simulink model "proyectomodelado"  (R2023a)
settings: Solver=ode15s  StartTime=0.0  StopTime=5.0  RelTol=1e-3
libraries: fl_lib x14, nesl_utility x6, slpidlib x1
settings Model: Creator=yosel  LastModifiedBy=nicol
settings DataIOCC: ReturnWorkspaceOutputs=off  TimeSaveName=t
settings DebuggingCC: AlgebraicLoopMsg=none

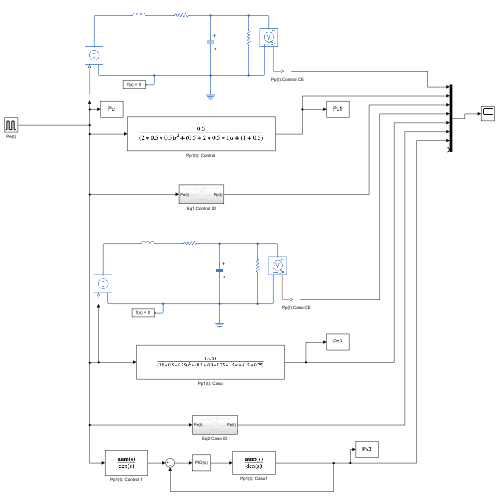
[thumbnail: Simulink's stored preview of the top-level diagram]
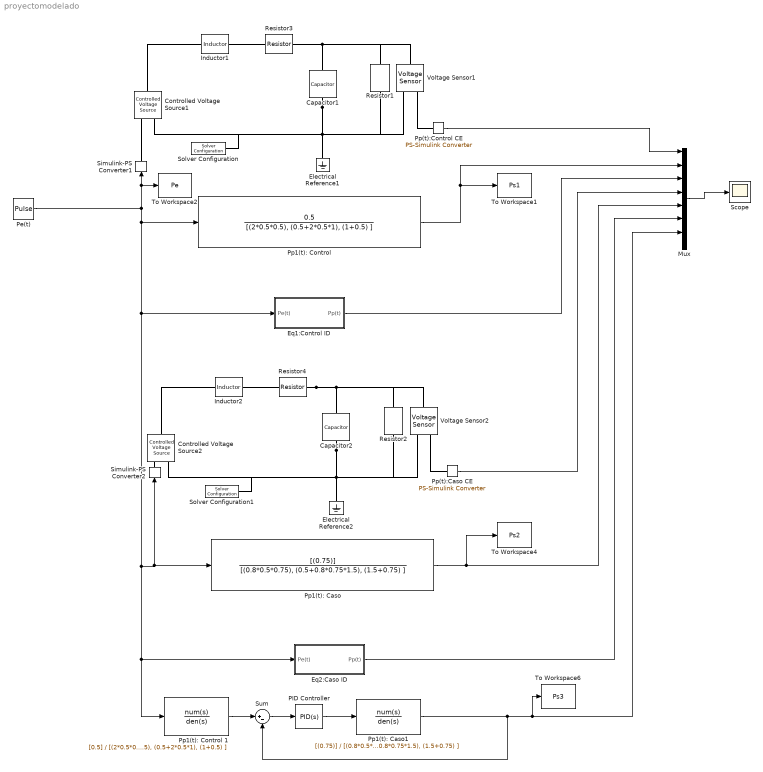
== system proyectomodelado ==
  Capacitor1 : fl_lib/Electrical/Electrical Elements/Capacitor  c=2 F  r=1e-6 Ohm  g=0 1/Ohm  i_specify=off  i_priority=None  i=0 A  i_nominal_specify=off  i_nominal_unit=A  i_nominal_value=1  v_specify=off  v_priority=None  v=0 V  v_nominal_specify=off  v_nominal_unit=V  v_nominal_value=1  vc_specify=off  vc_priority=High  vc=0 V  vc_nominal_specify=off  vc_nominal_unit=V  vc_nominal_value=1
  Capacitor2 : fl_lib/Electrical/Electrical Elements/Capacitor  c=0.8 F  r=1e-6 Ohm  g=0 1/Ohm  i_specify=off  i_priority=None  i=0 A  i_nominal_specify=off  i_nominal_unit=A  i_nominal_value=1  v_specify=off  v_priority=None  v=0 V  v_nominal_specify=off  v_nominal_unit=V  v_nominal_value=1  vc_specify=off  vc_priority=High  vc=0 V  vc_nominal_specify=off  vc_nominal_unit=V  vc_nominal_value=1
  Controlled Voltage Source1 : fl_lib/Electrical/Electrical Sources/Controlled Voltage Source
  Controlled Voltage Source2 : fl_lib/Electrical/Electrical Sources/Controlled Voltage Source
  Electrical Reference1 : fl_lib/Electrical/Electrical Elements/Electrical Reference
  Electrical Reference2 : fl_lib/Electrical/Electrical Elements/Electrical Reference
  Eq1:Control ID : Subsystem
  Eq2:Caso ID : Subsystem
  Inductor1 : fl_lib/Electrical/Electrical Elements/Inductor  l=0.5 H  r=0 Ohm  g=1e-9 1/Ohm  i_specify=off  i_priority=None  i=0 A  i_nominal_specify=off  i_nominal_unit=A  i_nominal_value=1  v_specify=off  v_priority=None  v=0 V  v_nominal_specify=off  v_nominal_unit=V  v_nominal_value=1  i_L_specify=off  i_L_priority=High  i_L=0 A  i_L_nominal_specify=off  i_L_nominal_unit=A  i_L_nominal_value=1
  Inductor2 : fl_lib/Electrical/Electrical Elements/Inductor  l=0.5 H  r=0 Ohm  g=1e-9 1/Ohm  i_specify=off  i_priority=None  i=0 A  i_nominal_specify=off  i_nominal_unit=A  i_nominal_value=1  v_specify=off  v_priority=None  v=0 V  v_nominal_specify=off  v_nominal_unit=V  v_nominal_value=1  i_L_specify=off  i_L_priority=High  i_L=0 A  i_L_nominal_specify=off  i_L_nominal_unit=A  i_L_nominal_value=1
  Mux : Mux  Inputs=8
  PID Controller : slpidlib/PID Controller  Controller=PID  Form=Parallel  TimeDomain=Continuous-time  UseExternalTs=off  SampleTime=-1  IntegratorMethod=Forward Euler  FilterMethod=Forward Euler  ControllerParametersSource=internal  P=2417168.60686299  I=213970849.102976  UseKiTs=off  D=6067.08740440942  N=1734073.08212751  UseFilter=on  TunerSelectOption=Transfer Function Based (PID Tuner App)  InitialConditionSource=internal  InitialConditionForIntegrator=0  InitialConditionForFilter=0  DifferentiatorICPrevScaledInput=0  ExternalReset=none  TrackingMode=off  Kt=1  LimitOutput=off  SatLimitsSource=internal  UpperSaturationLimit=inf  LowerSaturationLimit=-inf  LinearizeAsGain=on  AntiWindupMode=none  Kb=1  LimitIntegrator=off  UpperIntegratorSaturationLimit=inf  LowerIntegratorSaturationLimit=-inf  POutMin=[]  POutMax=[]  IOutMin=[]  IOutMax=[]  DOutMin=[]  DOutMax=[]  NOutMin=[]  NOutMax=[]  SumOutMin=[]  SumOutMax=[]  SaturationOutMin=[]  SaturationOutMax=[]  PParamMin=[]  PParamMax=[]  IParamMin=[]  IParamMax=[]  DParamMin=[]  DParamMax=[]  NParamMin=[]  NParamMax=[]  KbParamMin=[]  KbParamMax=[]  KtParamMin=[]  KtParamMax=[]  KbOutMin=[]  KbOutMax=[]  KtOutMin=[]  KtOutMax=[]  IntegratorOutMin=[]  IntegratorOutMax=[]  FilterOutMin=[]  FilterOutMax=[]  SumI1OutMin=[]  SumI1OutMax=[]  SumI2OutMin=[]  SumI2OutMax=[]  SumI3OutMin=[]  SumI3OutMax=[]  SumI4OutMin=[]  SumI4OutMax=[]  SumDOutMin=[]  SumDOutMax=[]  DifferentiatorOutMin=[]  DifferentiatorOutMax=[]  FilterDiffOutCoefMin=[]  FilterDiffOutCoefMax=[]  ReciprocalOutMin=[]  ReciprocalOutMax=[]  SumDenOutMin=[]  SumDenOutMax=[]  SumNumOutMin=[]  SumNumOutMax=[]  DivideOutMin=[]  DivideOutMax=[]  UdiffTsProdOutMin=[]  UdiffTsProdOutMax=[]  NTsProdOutMin=[]  NTsProdOutMax=[]  UintegralTsProdOutMin=[]  UintegralTsProdOutMax=[]  UngainTsProdOutMin=[]  UngainTsProdOutMax=[]  ClampingZeroOutDataTypeStr=Inherit: Inherit via back propagation  ClampingZeroOutMin=[]  ClampingZeroOutMax=[]  FilterDenConstantOutDataTypeStr=Inherit: Inherit via back propagation  FilterDenConstantOutMin=[]  FilterDenConstantOutMax=[]  PCopyOutDataTypeStr=Inherit: Inherit via back propagation  PCopyOutMin=[]  PCopyOutMax=[]  NCopyOutDataTypeStr=Inherit: Inherit via back propagation  NCopyOutMin=[]  NCopyOutMax=[]  IntegratorContinuousStateAttributes=''  IntegratorStateMustResolveToSignalObject=off  IntegratorRTWStateStorageClass=Auto  FilterContinuousStateAttributes=''  FilterStateMustResolveToSignalObject=off  FilterRTWStateStorageClass=Auto  ParallelPVariant=InternalParameters  IdealPVariant=Disabled  IVariant=InternalParameters  DVariant=InternalParameters  IntegratorVariant=Continuous  SatVariant=Disabled  AWVariant=Passthrough  PCopyVariant=Disabled  TRVariant=Disabled  FdbkBlocksVariant=Forward  IdealPFdbkVariant=Disabled  SatFdbkVariant=Disabled  DerivativeFilterVariant=ContFilter  NVariant=InternalParameters  NCopyVariant=Disabled  FilterICVariant=InternalICsFilter  IntegratorICVariant=InternalICs  ExternalResetVariant=Disabled  TRSumVariant=Passthrough  SumFdbkVariant=Disabled  SumVariant=Sum_PID  TsampFilterVariant=InternalTs  TsampNgainVariant=Passthrough  TsampIntegralVariant=Disabled_SignalSpec  ExternalSaturationOutDataTypeStr=Inherit: Same as second input
  Pe(t) : DiscretePulseGenerator  PulseType=Time based  Period=10  PulseWidth=5  PhaseDelay=1
  Pp(t):Caso CE : nesl_utility/PS-Simulink Converter  PhysicalDomain=network_engine_domain  SubClassName=ps_output  LeftPortType=input  RightPortType=output  PseudoPeriodic=off  Frequencies=[]  VectorFormat=1-D array  Unit=inherit  AffineConversion=off
  Pp(t):Control CE : nesl_utility/PS-Simulink Converter  PhysicalDomain=network_engine_domain  SubClassName=ps_output  LeftPortType=input  RightPortType=output  PseudoPeriodic=off  Frequencies=[]  VectorFormat=1-D array  Unit=inherit  AffineConversion=off
  Pp1(t): Caso : TransferFcn  Numerator=[(0.75)]  Denominator=[(0.8*0.5*0.75), (0.5+0.8*0.75*1.5), (1.5+0.75) ]
  Pp1(t): Caso1 : TransferFcn  Numerator=[(0.75)]  Denominator=[(0.8*0.5*0.75), (0.5+0.8*0.75*1.5), (1.5+0.75) ]
  "Pp1(t): Control " : TransferFcn  Numerator=[0.5]  Denominator=[(2*0.5*0.5), (0.5+2*0.5*1), (1+0.5) ]
  Pp1(t): Control 1 : TransferFcn  Numerator=[0.5]  Denominator=[(2*0.5*0.5), (0.5+2*0.5*1), (1+0.5) ]
  Resistor1 : fl_lib/Electrical/Electrical Elements/Resistor  R=0.5 Ohm  i_specify=off  i_priority=None  i=0 A  i_nominal_specify=off  i_nominal_unit=A  i_nominal_value=1  v_specify=off  v_priority=None  v=0 V  v_nominal_specify=off  v_nominal_unit=V  v_nominal_value=1
  Resistor2 : fl_lib/Electrical/Electrical Elements/Resistor  R=0.75 Ohm  i_specify=off  i_priority=None  i=0 A  i_nominal_specify=off  i_nominal_unit=A  i_nominal_value=1  v_specify=off  v_priority=None  v=0 V  v_nominal_specify=off  v_nominal_unit=V  v_nominal_value=1
  Resistor3 : fl_lib/Electrical/Electrical Elements/Resistor  R=1 Ohm  i_specify=off  i_priority=None  i=0 A  i_nominal_specify=off  i_nominal_unit=A  i_nominal_value=1  v_specify=off  v_priority=None  v=0 V  v_nominal_specify=off  v_nominal_unit=V  v_nominal_value=1
  Resistor4 : fl_lib/Electrical/Electrical Elements/Resistor  R=1.5 Ohm  i_specify=off  i_priority=None  i=0 A  i_nominal_specify=off  i_nominal_unit=A  i_nominal_value=1  v_specify=off  v_priority=None  v=0 V  v_nominal_specify=off  v_nominal_unit=V  v_nominal_value=1
  Scope : Scope
  Simulink-PS Converter1 : nesl_utility/Simulink-PS Converter  PhysicalDomain=network_engine_domain  SubClassName=ps_input  LeftPortType=input  RightPortType=output  PseudoPeriodic=off  Frequencies=[]  NoiseDistribution=none  NoiseParameters=[]  Unit=1  AffineConversion=off  FilteringAndDerivatives=provide  SimscapeFilterOrder=1  InputFilterTimeConstant=0.001  UdotUserProvided=0
  Simulink-PS Converter2 : nesl_utility/Simulink-PS Converter  PhysicalDomain=network_engine_domain  SubClassName=ps_input  LeftPortType=input  RightPortType=output  PseudoPeriodic=off  Frequencies=[]  NoiseDistribution=none  NoiseParameters=[]  Unit=1  AffineConversion=off  FilteringAndDerivatives=provide  SimscapeFilterOrder=1  InputFilterTimeConstant=0.001  UdotUserProvided=0
  Solver Configuration : nesl_utility/Solver Configuration  PhysicalDomain=network_engine_domain  SubClassName=solver  LeftPortType=input  RightPortType=generic  Tones=[]  Harmonics=[]  SimulateNoise=off  Profile=off  UseLocalSampling=off  EnableSwitchedLinearOptims=on  FrequencyDomain=off  UseCCode=off  RelTol=0.001  AbsTol=0.001  MinStep=1e-09  ToWorkspace=off  RevertToSquareIcSolve=off  NumHomotopyIterations=100  PhasorMode=off  PhasorModeNumHarmonics=1  ConsistencySolver=NEWTON_XTOL_AFTER_FTOL  IndexReductionMethod=DerivativeReplacement  DoDC=off  ResidualTolerance=1e-09  ConsistencyTolSource=GLOBAL  ConsistencyAbsTol=0.001  ConsistencyRelTol=0.001  ConsistencyTolFactor=0.001  UseLocalSolver=off  LocalSolverChoice=NE_BACKWARD_EULER_ADVANCER  ResolveIndetEquations=on  FunctionEvalNumThread=1  LocalSolverSampleTime=0.001  DoFixedCost=off  MaxNonlinIter=3  MaxModeIter=2  ComputeImpulses=off  ImpulseIterations=2  LinearAlgebra=auto  LinearAlgebraNumThread=0  EquationFormulation=NE_TIME_EF  DelaysMemoryBudget=1024  AutomaticFiltering=on  FilteringTimeConstant=0.001  PartitionStorageMethod=AS_NEEDED  PartitionMemoryBudget=1024  PartitionMethod=ROBUST
  Solver Configuration1 : nesl_utility/Solver Configuration  PhysicalDomain=network_engine_domain  SubClassName=solver  LeftPortType=input  RightPortType=generic  Tones=[]  Harmonics=[]  SimulateNoise=off  Profile=off  UseLocalSampling=off  EnableSwitchedLinearOptims=on  FrequencyDomain=off  UseCCode=off  RelTol=0.001  AbsTol=0.001  MinStep=1e-09  ToWorkspace=off  RevertToSquareIcSolve=off  NumHomotopyIterations=100  PhasorMode=off  PhasorModeNumHarmonics=1  ConsistencySolver=NEWTON_XTOL_AFTER_FTOL  IndexReductionMethod=DerivativeReplacement  DoDC=off  ResidualTolerance=1e-09  ConsistencyTolSource=GLOBAL  ConsistencyAbsTol=0.001  ConsistencyRelTol=0.001  ConsistencyTolFactor=0.001  UseLocalSolver=off  LocalSolverChoice=NE_BACKWARD_EULER_ADVANCER  ResolveIndetEquations=on  FunctionEvalNumThread=1  LocalSolverSampleTime=0.001  DoFixedCost=off  MaxNonlinIter=3  MaxModeIter=2  ComputeImpulses=off  ImpulseIterations=2  LinearAlgebra=auto  LinearAlgebraNumThread=0  EquationFormulation=NE_TIME_EF  DelaysMemoryBudget=1024  AutomaticFiltering=on  FilteringTimeConstant=0.001  PartitionStorageMethod=AS_NEEDED  PartitionMemoryBudget=1024  PartitionMethod=ROBUST
  Sum : Sum  Inputs=|+-
  To Workspace1 : ToWorkspace  VariableName=Ps1  SampleTime=-1
  To Workspace2 : ToWorkspace  VariableName=Pe  SampleTime=-1
  To Workspace4 : ToWorkspace  VariableName=Ps2  SampleTime=-1
  To Workspace6 : ToWorkspace  VariableName=Ps3  SampleTime=-1
  Voltage Sensor1 : fl_lib/Electrical/Electrical Sensors/Voltage Sensor
  Voltage Sensor2 : fl_lib/Electrical/Electrical Sensors/Voltage Sensor
  wires:
  Mux/1 -> Scope/1
  "Pp1(t): Control "/1 -> To Workspace1/1, Mux/2
  Pp(t):Control CE/1 -> Mux/1
  Pe(t)/1 -> To Workspace2/1, Simulink-PS Converter1/1, Eq1:Control ID/1(Pe(t)), Pp1(t): Control 1/1, Eq2:Caso ID/1(Pe(t)), Simulink-PS Converter2/1, Pp1(t): Caso/1, "Pp1(t): Control "/1
  Pp1(t): Control 1/1 -> Sum/1
  Sum/1 -> PID Controller/1
  PID Controller/1 -> Pp1(t): Caso1/1
  Pp1(t): Caso1/1 -> Sum/2, To Workspace6/1, Mux/7
  Eq1:Control ID/1(Pp(t)) -> Mux/3
  Pp(t):Caso CE/1 -> Mux/4
  Pp1(t): Caso/1 -> To Workspace4/1, Mux/5
  Eq2:Caso ID/1(Pp(t)) -> Mux/6
  connections:
  Inductor1/LConn1 -- Controlled Voltage Source1/LConn1
  Capacitor1/RConn1 -- Voltage Sensor1/RConn2 -- Resistor1/LConn1 -- Solver Configuration/RConn1 -- Controlled Voltage Source1/RConn2 -- Electrical Reference1/LConn1
  Capacitor1/LConn1 -- Voltage Sensor1/LConn1 -- Resistor1/RConn1 -- Resistor3/LConn1
  Voltage Sensor1/RConn1 -- Pp(t):Control CE/LConn1
  Inductor1/RConn1 -- Resistor3/RConn1
  Simulink-PS Converter1/RConn1 -- Controlled Voltage Source1/RConn1
  Resistor4/LConn1 -- Capacitor2/LConn1 -- Voltage Sensor2/LConn1 -- Resistor2/RConn1
  Capacitor2/RConn1 -- Voltage Sensor2/RConn2 -- Resistor2/LConn1 -- Solver Configuration1/RConn1 -- Controlled Voltage Source2/RConn2 -- Electrical Reference2/LConn1
  Inductor2/LConn1 -- Controlled Voltage Source2/LConn1
  Voltage Sensor2/RConn1 -- Pp(t):Caso CE/LConn1
  Inductor2/RConn1 -- Resistor4/RConn1
  Simulink-PS Converter2/RConn1 -- Controlled Voltage Source2/RConn1

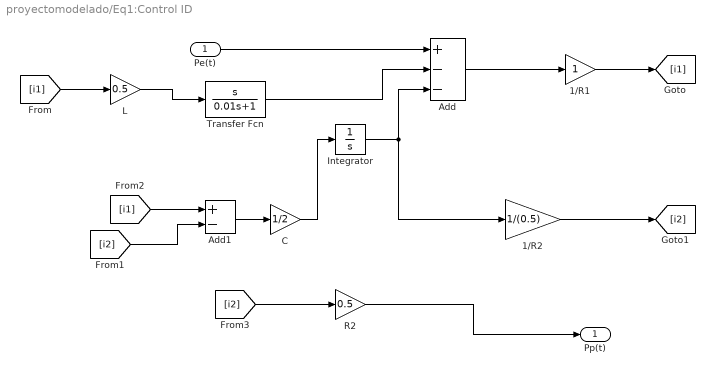
== system proyectomodelado/Eq1:Control ID ==
  Pe(t) : Inport
  1/R1 : Gain
  1/R2 : Gain  Gain=1/(0.5)
  Add : Sum  Inputs=+--
  Add1 : Sum  Inputs=+-
  C : Gain  Gain=1/2
  Integrator : Integrator
  L : Gain  Gain=0.5
  R2 : Gain  Gain=0.5
  Transfer Fcn : TransferFcn  Numerator=[1 0]  Denominator=[0.01 1]
  Pp(t) : Outport
  wires:
  Pe(t)/1 -> Add/1
  Add/1 -> 1/R1/1
  1/R1/1 -> [i1]
  [i1] -> L/1
  [i1] -> Add1/1
  [i2] -> Add1/2
  Add1/1 -> C/1
  C/1 -> Integrator/1
  Integrator/1 -> 1/R2/1, Add/3
  1/R2/1 -> [i2]
  R2/1 -> Pp(t)/1
  [i2] -> R2/1
  L/1 -> Transfer Fcn/1
  Transfer Fcn/1 -> Add/2

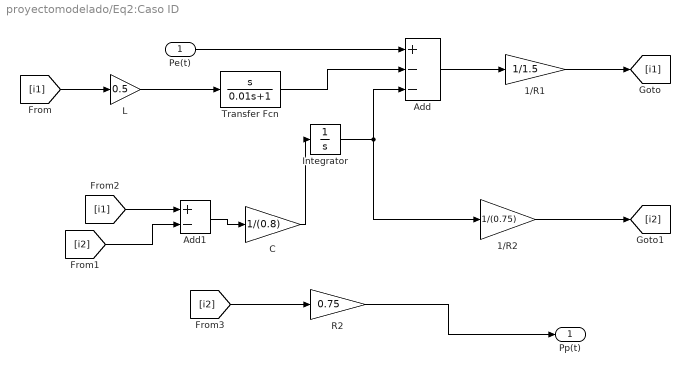
== system proyectomodelado/Eq2:Caso ID ==
  Pe(t) : Inport
  1/R1 : Gain  Gain=1/1.5
  1/R2 : Gain  Gain=1/(0.75)
  Add : Sum  Inputs=+--
  Add1 : Sum  Inputs=+-
  C : Gain  Gain=1/(0.8)
  Integrator : Integrator
  L : Gain  Gain=0.5
  R2 : Gain  Gain=0.75
  Transfer Fcn : TransferFcn  Numerator=[1 0]  Denominator=[0.01 1]
  Pp(t) : Outport
  wires:
  Pe(t)/1 -> Add/1
  Add/1 -> 1/R1/1
  1/R1/1 -> [i1]
  [i1] -> L/1
  [i1] -> Add1/1
  [i2] -> Add1/2
  Add1/1 -> C/1
  C/1 -> Integrator/1
  Integrator/1 -> 1/R2/1, Add/3
  1/R2/1 -> [i2]
  R2/1 -> Pp(t)/1
  [i2] -> R2/1
  L/1 -> Transfer Fcn/1
  Transfer Fcn/1 -> Add/2
